simulink model "Direct_Motor_Function"  (Simulink 7.5)
settings: Solver=ode45  StartTime=0.0  StopTime=10.0  RelTol=1e-3
settings Model: Creator=lm  LastModifiedBy=lm

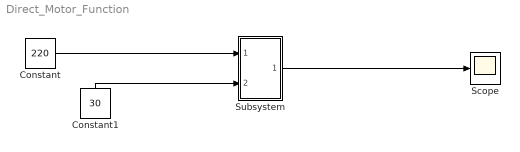
== system Direct_Motor_Function ==
  Constant : Constant  Value=220  OutDataType=fixdt(1, 16)  OutScaling=2^0
  Constant1 : Constant  Value=30  OutDataType=fixdt(1, 16)  OutScaling=2^0
  Scope : Scope
  Subsystem : Subsystem
  wires:
  Constant/1 -> Subsystem/1(In1)
  Subsystem/1(Out1) -> Scope/1
  Constant1/1 -> Subsystem/2(In2)

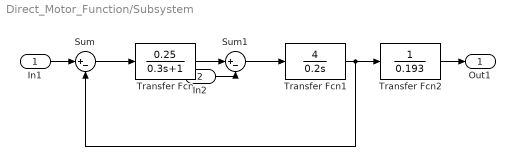
== system Direct_Motor_Function/Subsystem ==
  In1 : Inport
  In2 : Inport  Port=2
  Sum : Sum  Inputs=|+-  OutDataType=fixdt(1, 16)  OutScaling=2^0
  Sum1 : Sum  Inputs=|+-  OutDataType=fixdt(1, 16)  OutScaling=2^0
  Transfer Fcn : TransferFcn  Numerator=0.25  Denominator=[0.3 1]
  Transfer Fcn1 : TransferFcn  Numerator=4  Denominator=[0.2 0]
  Transfer Fcn2 : TransferFcn  Numerator=1  Denominator=[0 0.193]
  Out1 : Outport
  wires:
  Sum/1 -> Transfer Fcn/1
  Transfer Fcn/1 -> Sum1/1
  Sum1/1 -> Transfer Fcn1/1
  Transfer Fcn1/1 -> Transfer Fcn2/1, Sum/2
  In1/1 -> Sum/1
  Transfer Fcn2/1 -> Out1/1
  In2/1 -> Sum1/2
